simulink model "DBX_model_all"  (R2015a)
settings: Solver=ode2  SolverMode=SingleTasking  StartTime=0.0  StopTime=10  FixedStep=T_sim  RelTol=1e-3
undefined symbols (not defined in the file or in its folder): A_M, Alpha_unique_rad, as, B_span, Beta_unique_rad, C_D_q, C_l, C_l_delta_a_Asim, C_l_delta_rv_Asim, C_l_p, C_l_r, C_Lift_q, C_m, C_m_q, C_n, C_n_delta_a_Asim, C_n_delta_rv_Asim, C_n_p, C_n_r, C_X, C_Y, C_Y_delta_rv_Asim, C_Y_p, C_Y_r, C_Z, CG, CMA, DBX_aero, DBX_aero_param, delta_elev_unique_rad, DOWN_0, EAST_0, F, g, h_1, h_2, h_3, I_BAC, Initial_Omegas, Initial_Torques, Ion, L_M, Lithium, m, MIL, NORTH_0, P_0, Q_0, R_0, Rotation_sign, Servo_calib, T_sim, U_0, V_0, W_0
libraries: simulink x19, DBX_model x14, aerolibwind2 x12, aerolibasang x9, aerolibadyn x4, aerolibatmos2 x2, powerlib x2, aerolibtransform2 x1, electricdrivelib x1
(part 3 of 3)

== system DBX_model_all/Aeromodel/Aero model V2 parametric/Aerodynamics/Moment Coefficients/C_m_T ==
  note: Deflexiones del modelo Aero:
      |
      | delta_ail
      | delta_elev
      | delta_rudder
  alpha : Inport
  beta : Inport  Port=2
  body_rates_adim : Inport  Port=3  PortDimensions=[3 1]
  defl_control : Inport  Port=4
  Add : Sum  Inputs=+++|
  C_m : Subsystem
  C_m_delta_elev : Subsystem
  C_m_q : Constant  Value=DBX_aero_param.C_m_q
  Divide : Product  Inputs=**
  Selector : Selector  InputPortWidth=3  Indices=2
  Selector2 : Selector  InputPortWidth=3  Indices=2
  C_m_T : Outport
  wires:
  Add/1 -> C_m_T/1
  C_m/1(C_m_out) -> Add/1
  Divide/1 -> Add/3
  defl_control/1 -> Selector2/1
  body_rates_adim/1 -> Selector/1
  C_m_q/1 -> Divide/2
  Selector/1 -> Divide/1
  beta/1 -> C_m/2(y)
  alpha/1 -> C_m_delta_elev/1(x), C_m/1(x)
  Selector2/1 -> C_m_delta_elev/2(y)
  C_m_delta_elev/1(C_m_delta_elev_out) -> Add/2

== system DBX_model_all/Aeromodel/Aero model V2 parametric/Aerodynamics/Moment Coefficients/C_n_T ==
  note: Deflexiones del modelo Aero:
      |
      | delta_ail
      | delta_elev
      | delta_rudder
  alpha : Inport
  beta : Inport  Port=2
  body_rates_adim : Inport  Port=3  PortDimensions=[3 1]
  defl_control : Inport  Port=4
  Add : Sum  Inputs=+++++
  C_n : Subsystem
  C_n_delta_a : Constant  Value=DBX_aero_param.C_n_delta_ale
  C_n_delta_rudd : Constant  Value=DBX_aero_param.C_n_delta_rud
  C_n_p : Constant  Value=DBX_aero_param.C_n_p
  C_n_r : Constant  Value=DBX_aero_param.C_n_r
  Divide{,1..3} (4 alike) : Product  Inputs=**
  Selector : Selector  InputPortWidth=3  Indices=3
  Selector1 : Selector  InputPortWidth=3  Indices=3
  Selector2 : Selector  InputPortWidth=3
  Selector3 : Selector  InputPortWidth=3
  C_n_T : Outport
  wires:
  Divide1/1 -> Add/5
  Divide2/1 -> Add/4
  Divide3/1 -> Add/3
  Divide/1 -> Add/2
  C_n/1(C_n_out) -> Add/1
  Selector/1 -> Divide/1
  C_n_p/1 -> Divide3/2
  Selector3/1 -> Divide3/1
  body_rates_adim/1 -> Selector/1, Selector3/1
  C_n_r/1 -> Divide/2
  Selector1/1 -> Divide1/1
  C_n_delta_rudd/1 -> Divide1/2
  Selector2/1 -> Divide2/1
  C_n_delta_a/1 -> Divide2/2
  defl_control/1 -> Selector2/1, Selector1/1
  Add/1 -> C_n_T/1
  beta/1 -> C_n/2(y)
  alpha/1 -> C_n/1(x)

== system DBX_model_all/Aeromodel/Aero model V2 parametric/Aerodynamics/Wind-axes Velocities/Calculate alphadot ==
  note: W
  note: Calculate alphadot
  "[Udot Vdot Wdot]" : Inport
  "[U V W]" : Inport  Port=2
  Demux : Demux  Outputs=3
  Demux1 : Demux  Outputs=3
  Math Function : Math  Operator=square  SaturateOnIntegerOverflow=on
  Math Function1 : Math  Operator=square  SaturateOnIntegerOverflow=on
  Product : Product  RndMeth=Zero
  Product1 : Product  RndMeth=Zero
  Product2 : Product  Inputs=*/  RndMeth=Zero
  Sum : Sum  Inputs=-|+
  Sum1 : Sum  Inputs=+|+
  Terminator : Terminator
  Terminator1 : Terminator
  alphadot : Outport
  wires:
  Demux/1 -> Product1/1  "Udot"
  Demux/3 -> Product/1  "Wdot"
  Demux/2 -> Terminator/1
  Demux1/1 -> Product/2, Math Function/1  "U"
  Demux1/3 -> Product1/2, Math Function1/1
  Math Function/1 -> Sum1/1
  Math Function1/1 -> Sum1/2
  Sum1/1 -> Product2/2  "U^2 + W^2"
  Product1/1 -> Sum/1  "W Udot"
  Product/1 -> Sum/2  "U Wdot"
  Sum/1 -> Product2/1
  Demux1/2 -> Terminator1/1
  "[U V W]"/1 -> Demux1/1
  "[Udot Vdot Wdot]"/1 -> Demux/1
  Product2/1 -> alphadot/1  "alphadot"

== system DBX_model_all/Aeromodel/Aero model aerosonde/Aerodynamics/Force Coefficients/Drag Coefficients ==
  note: Drag coefficient
  control : Inport
  Mach : Inport  Port=2
  CL : Inport  Port=3  PortDimensions=1
  (CL-CL0)^2/(pi e AR) : Gain  Gain=1/as.pieaR  Multiplication=Matrix(K*u)  SaturateOnIntegerOverflow=on  OutDataTypeStr=Inherit: Same as input  ParamDataTypeStr=Inherit: Same as input
  Abs4 : Abs  SaturateOnIntegerOverflow=on
  CDM : Gain  Gain=as.CDM  SaturateOnIntegerOverflow=on  OutDataTypeStr=Inherit: Same as input  ParamDataTypeStr=Inherit: Same as input
  CDdf : Gain  Gain=[as.CDdf, as.CDde, as.CDda, as.CDdr]  Multiplication=Matrix(K*u)  SaturateOnIntegerOverflow=on  OutDataTypeStr=Inherit: Same as input  ParamDataTypeStr=Inherit: Same as input
  CL min drag : Constant  Value=as.CLmind
  CL^2 : Math  Operator=square  SaturateOnIntegerOverflow=on
  Constant terms : Constant  Value=as.CD0
  Sum : Sum  Inputs=|+-  SaturateOnIntegerOverflow=on  InputSameDT=on  OutDataTypeStr=Inherit: Same as first input
  Sum1 : Sum  Inputs=++++  SaturateOnIntegerOverflow=on  InputSameDT=on  OutDataTypeStr=Inherit: Same as first input
  CD : Outport
  wires:
  (CL-CL0)^2/(pi e AR)/1 -> Sum1/4
  CL min drag/1 -> Sum/2
  CL/1 -> Sum/1
  Sum/1 -> CL^2/1
  CL^2/1 -> (CL-CL0)^2/(pi e AR)/1
  Sum1/1 -> CD/1  "CD"
  Mach/1 -> CDM/1
  control/1 -> Abs4/1
  Abs4/1 -> CDdf/1
  CDM/1 -> Sum1/3
  CDdf/1 -> Sum1/2
  Constant terms/1 -> Sum1/1

== system DBX_model_all/Aeromodel/Aero model aerosonde/Aerodynamics/Force Coefficients/Lift Coefficients ==
  note: Lift Coefficients
  alpha : Inport
  control : Inport  Port=2
  alphadot : Inport  Port=3
  pqr : Inport  Port=4
  2V_a : Inport  Port=5
  Mach : Inport  Port=6
  CL*c/(2V_a) : Product  Inputs=*/  SaturateOnIntegerOverflow=on  InputSameDT=on  OutDataTypeStr=Inherit: Same as first input
  CL0 : Constant  Value=as.CL0
  CLM : Gain  Gain=as.CLM  SaturateOnIntegerOverflow=on  OutDataTypeStr=Inherit: Same as input  ParamDataTypeStr=Inherit: Same as input
  CLalpha : Gain  Gain=as.CLalpha  SaturateOnIntegerOverflow=on  OutDataTypeStr=Inherit: Same as input  ParamDataTypeStr=Inherit: Same as input
  CLalphadot : Gain  Gain=as.CLalphadot  Multiplication=Matrix(K*u)  SaturateOnIntegerOverflow=on  OutDataTypeStr=Inherit: Same as input  ParamDataTypeStr=Inherit: Same as input
  CLq : Gain  Gain=[0, as.CLq, 0]  Multiplication=Matrix(K*u)  SaturateOnIntegerOverflow=on  OutDataTypeStr=Inherit: Same as input  ParamDataTypeStr=Inherit: Same as input
  Sum : Sum  SaturateOnIntegerOverflow=on  InputSameDT=on  OutDataTypeStr=Inherit: Same as first input
  Sum2 : Sum  Inputs=+++++  SaturateOnIntegerOverflow=on  InputSameDT=on  OutDataTypeStr=Inherit: Same as first input
  "[CLdf, CLde, 0, 0]" : Gain  Gain=[as.CLdf, as.CLde, 0, 0]  Multiplication=Matrix(K*u)  SaturateOnIntegerOverflow=on  OutDataTypeStr=Inherit: Same as input  ParamDataTypeStr=Inherit: Same as input
  c : Gain  Gain=as.c  SaturateOnIntegerOverflow=on  OutDataTypeStr=Inherit: Same as input  ParamDataTypeStr=Inherit: Same as input
  CL : Outport
  wires:
  alphadot/1 -> CLalphadot/1
  alpha/1 -> CLalpha/1
  Mach/1 -> CLM/1
  2V_a/1 -> CL*c/(2V_a)/2
  pqr/1 -> CLq/1
  control/1 -> "[CLdf, CLde, 0, 0]"/1
  c/1 -> CL*c/(2V_a)/1
  CL*c/(2V_a)/1 -> Sum2/4
  CLM/1 -> Sum2/5
  Sum2/1 -> CL/1  "CL"
  "[CLdf, CLde, 0, 0]"/1 -> Sum2/3
  CLalpha/1 -> Sum2/2
  CL0/1 -> Sum2/1
  Sum/1 -> c/1
  CLalphadot/1 -> Sum/1
  CLq/1 -> Sum/2

== system DBX_model_all/Aeromodel/Aero model aerosonde/Aerodynamics/Force Coefficients/Side Force Coefficients ==
  note: Side force coefficients
  beta : Inport
  control : Inport  Port=2
  angular rates : Inport  Port=3
  2V_a : Inport  Port=4
  CY*b/(2V_a) : Product  Inputs=*/  SaturateOnIntegerOverflow=on  InputSameDT=on  OutDataTypeStr=Inherit: Same as first input
  CYbeta : Gain  Gain=as.CYbeta  SaturateOnIntegerOverflow=on  OutDataTypeStr=Inherit: Same as input  ParamDataTypeStr=Inherit: Same as input
  Sum3 : Sum  Inputs=+++  SaturateOnIntegerOverflow=on  InputSameDT=on  OutDataTypeStr=Inherit: Same as first input
  Wing span1 : Gain  Gain=as.b  SaturateOnIntegerOverflow=on  OutDataTypeStr=Inherit: Same as input  ParamDataTypeStr=Inherit: Same as input
  "[0, 0, CYda, CYdr]" : Gain  Gain=[0, 0, as.CYda, as.CYdr]  Multiplication=Matrix(K*u)  SaturateOnIntegerOverflow=on  OutDataTypeStr=Inherit: Same as input  ParamDataTypeStr=Inherit: Same as input
  "[CYp, 0, CYr]" : Gain  Gain=[as.CYp, 0, as.CYr]  Multiplication=Matrix(K*u)  SaturateOnIntegerOverflow=on  OutDataTypeStr=Inherit: Same as input  ParamDataTypeStr=Inherit: Same as input
  CY : Outport
  wires:
  beta/1 -> CYbeta/1
  2V_a/1 -> CY*b/(2V_a)/2
  angular rates/1 -> "[CYp, 0, CYr]"/1
  control/1 -> "[0, 0, CYda, CYdr]"/1
  Wing span1/1 -> CY*b/(2V_a)/1
  Sum3/1 -> CY/1  "CY"
  CY*b/(2V_a)/1 -> Sum3/3
  "[0, 0, CYda, CYdr]"/1 -> Sum3/2
  CYbeta/1 -> Sum3/1
  "[CYp, 0, CYr]"/1 -> Wing span1/1

== system DBX_model_all/Aeromodel/Aero model aerosonde/Aerodynamics/Moment Coefficients/Pitch Moment Coefficients ==
  alpha : Inport
  control : Inport  Port=2
  alphadot : Inport  Port=3
  pqr : Inport  Port=4
  2V_a : Inport  Port=5
  Mach : Inport  Port=6
  CMalpha : Gain  Gain=as.Cmalpha  SaturateOnIntegerOverflow=on  OutDataTypeStr=Inherit: Same as input  ParamDataTypeStr=Inherit: Same as input
  Cm*c/(2V_a) : Product  Inputs=*/  SaturateOnIntegerOverflow=on  InputSameDT=on  OutDataTypeStr=Inherit: Same as first input
  Cm0 : Constant  Value=as.Cm0
  CmM : Gain  Gain=as.CmM  SaturateOnIntegerOverflow=on  OutDataTypeStr=Inherit: Same as input  ParamDataTypeStr=Inherit: Same as input
  Cmalphadot : Gain  Gain=as.Cmalphadot  Multiplication=Matrix(K*u)  SaturateOnIntegerOverflow=on  OutDataTypeStr=Inherit: Same as input  ParamDataTypeStr=Inherit: Same as input
  Cmq : Gain  Gain=[0, as.Cmq, 0]  Multiplication=Matrix(K*u)  SaturateOnIntegerOverflow=on  OutDataTypeStr=Inherit: Same as input  ParamDataTypeStr=Inherit: Same as input
  Sum : Sum  SaturateOnIntegerOverflow=on  InputSameDT=on  OutDataTypeStr=Inherit: Same as first input
  Sum2 : Sum  Inputs=+++++  SaturateOnIntegerOverflow=on  InputSameDT=on  OutDataTypeStr=Inherit: Same as first input
  "[Cmdf, Cmde, 0, 0]" : Gain  Gain=[as.Cmdf, as.Cmde, 0, 0]  Multiplication=Matrix(K*u)  SaturateOnIntegerOverflow=on  OutDataTypeStr=Inherit: Same as input  ParamDataTypeStr=Inherit: Same as input
  c : Gain  Gain=as.c  SaturateOnIntegerOverflow=on  OutDataTypeStr=Inherit: Same as input  ParamDataTypeStr=Inherit: Same as input
  Cm : Outport
  wires:
  Cmq/1 -> Sum/2
  Cmalphadot/1 -> Sum/1
  Sum/1 -> c/1
  Cm0/1 -> Sum2/1
  CMalpha/1 -> Sum2/2
  "[Cmdf, Cmde, 0, 0]"/1 -> Sum2/3
  Sum2/1 -> Cm/1  "Cm"
  CmM/1 -> Sum2/5
  Cm*c/(2V_a)/1 -> Sum2/4
  c/1 -> Cm*c/(2V_a)/1
  control/1 -> "[Cmdf, Cmde, 0, 0]"/1
  pqr/1 -> Cmq/1
  2V_a/1 -> Cm*c/(2V_a)/2
  Mach/1 -> CmM/1
  alpha/1 -> CMalpha/1
  alphadot/1 -> Cmalphadot/1

== system DBX_model_all/Aeromodel/Aero model aerosonde/Aerodynamics/Moment Coefficients/Roll Moment Coefficients ==
  note: Roll moment coefficient
  beta : Inport
  control : Inport  Port=2
  angular rates : Inport  Port=3
  2V : Inport  Port=4
  CY*b/(2V) : Product  Inputs=*/  SaturateOnIntegerOverflow=on  InputSameDT=on  OutDataTypeStr=Inherit: Same as first input
  Clbeta : Gain  Gain=as.Clbeta  SaturateOnIntegerOverflow=on  OutDataTypeStr=Inherit: Same as input  ParamDataTypeStr=Inherit: Same as input
  Sum3 : Sum  Inputs=+++  SaturateOnIntegerOverflow=on  InputSameDT=on  OutDataTypeStr=Inherit: Same as first input
  Wing span : Gain  Gain=as.b  SaturateOnIntegerOverflow=on  OutDataTypeStr=Inherit: Same as input  ParamDataTypeStr=Inherit: Same as input
  "[0, 0, Clda, Cldr]" : Gain  Gain=[0, 0, as.Clda, as.Cldr]  Multiplication=Matrix(K*u)  SaturateOnIntegerOverflow=on  OutDataTypeStr=Inherit: Same as input  ParamDataTypeStr=Inherit: Same as input
  "[Clp, 0, Clr]" : Gain  Gain=[as.Clp, 0, as.Clr]  Multiplication=Matrix(K*u)  SaturateOnIntegerOverflow=on  OutDataTypeStr=Inherit: Same as input  ParamDataTypeStr=Inherit: Same as input
  Cl : Outport
  wires:
  "[Clp, 0, Clr]"/1 -> Wing span/1
  Clbeta/1 -> Sum3/1
  "[0, 0, Clda, Cldr]"/1 -> Sum3/2
  CY*b/(2V)/1 -> Sum3/3
  Sum3/1 -> Cl/1  "Cl"
  Wing span/1 -> CY*b/(2V)/1
  control/1 -> "[0, 0, Clda, Cldr]"/1
  angular rates/1 -> "[Clp, 0, Clr]"/1
  2V/1 -> CY*b/(2V)/2
  beta/1 -> Clbeta/1

== system DBX_model_all/Aeromodel/Aero model aerosonde/Aerodynamics/Moment Coefficients/Yaw Moment Coefficients ==
  note: Yaw moment coefficient
  beta : Inport
  control : Inport  Port=2
  angular rates : Inport  Port=3
  2V_a : Inport  Port=4
  Cn*b/(2V_a) : Product  Inputs=*/  SaturateOnIntegerOverflow=on  InputSameDT=on  OutDataTypeStr=Inherit: Same as first input
  Cnbeta : Gain  Gain=as.Cnbeta  SaturateOnIntegerOverflow=on  OutDataTypeStr=Inherit: Same as input  ParamDataTypeStr=Inherit: Same as input
  Sum3 : Sum  Inputs=+++  SaturateOnIntegerOverflow=on  InputSameDT=on  OutDataTypeStr=Inherit: Same as first input
  Wing span : Gain  Gain=as.b  SaturateOnIntegerOverflow=on  OutDataTypeStr=Inherit: Same as input  ParamDataTypeStr=Inherit: Same as input
  "[0, 0, Cnda, Cndr]" : Gain  Gain=[0, 0, as.Cnda, as.Cndr]  Multiplication=Matrix(K*u)  SaturateOnIntegerOverflow=on  OutDataTypeStr=Inherit: Same as input  ParamDataTypeStr=Inherit: Same as input
  "[Cnp, 0, Cnr]" : Gain  Gain=[as.Cnp, 0, as.Cnr]  Multiplication=Matrix(K*u)  SaturateOnIntegerOverflow=on  OutDataTypeStr=Inherit: Same as input  ParamDataTypeStr=Inherit: Same as input
  Cn : Outport
  wires:
  beta/1 -> Cnbeta/1
  2V_a/1 -> Cn*b/(2V_a)/2
  angular rates/1 -> "[Cnp, 0, Cnr]"/1
  control/1 -> "[0, 0, Cnda, Cndr]"/1
  Wing span/1 -> Cn*b/(2V_a)/1
  Sum3/1 -> Cn/1  "Cn"
  Cn*b/(2V_a)/1 -> Sum3/3
  "[0, 0, Cnda, Cndr]"/1 -> Sum3/2
  Cnbeta/1 -> Sum3/1
  "[Cnp, 0, Cnr]"/1 -> Wing span/1

== system DBX_model_all/Aeromodel/Aero model aerosonde/Aerodynamics/Wind-axes Velocities/Calculate alphadot ==
  note: Calculate alphadot
  note: W
  "[Udot Vdot Wdot]" : Inport
  "[U V W]" : Inport  Port=2
  Demux : Demux  Outputs=3
  Demux1 : Demux  Outputs=3
  Math Function : Math  Operator=square  SaturateOnIntegerOverflow=on
  Math Function1 : Math  Operator=square  SaturateOnIntegerOverflow=on
  Product : Product  RndMeth=Zero
  Product1 : Product  RndMeth=Zero
  Product2 : Product  Inputs=*/  RndMeth=Zero
  Sum : Sum  Inputs=-|+
  Sum1 : Sum  Inputs=+|+
  Terminator : Terminator
  Terminator1 : Terminator
  alphadot : Outport
  wires:
  Product2/1 -> alphadot/1  "alphadot"
  "[Udot Vdot Wdot]"/1 -> Demux/1
  "[U V W]"/1 -> Demux1/1
  Demux1/2 -> Terminator1/1
  Sum/1 -> Product2/1
  Product/1 -> Sum/2  "U Wdot"
  Product1/1 -> Sum/1  "W Udot"
  Sum1/1 -> Product2/2  "U^2 + W^2"
  Math Function1/1 -> Sum1/2
  Math Function/1 -> Sum1/1
  Demux1/3 -> Math Function1/1, Product1/2
  Demux1/1 -> Math Function/1, Product/2  "U"
  Demux/2 -> Terminator/1
  Demux/3 -> Product/1  "Wdot"
  Demux/1 -> Product1/1  "Udot"

== system DBX_model_all/Aeromodel/Aero model V2 parametric/Aerodynamics/Force Coefficients/C_X_T/C_X ==
  x : Inport
  y : Inport  Port=2
  C_X : MATLAB Function
  Constant : Constant  Value=DBX_aero_param.C_X.a
  Constant1 : Constant  Value=DBX_aero_param.C_X.x_lim
  Constant2 : Constant  Value=DBX_aero_param.C_X.y_lim
  Demux : Demux  Outputs=2
  Demux1 : Demux  Outputs=2
  Saturation Dynamic : simulink/Discontinuities/Saturation Dynamic  OutMin=[]  OutMax=[]  OutDataTypeStr=Inherit: Same as second input  OutDataType=fixdt(1, 16)  OutScaling=2^-10  DoSatur=off
  Saturation Dynamic1 : simulink/Discontinuities/Saturation Dynamic  OutMin=[]  OutMax=[]  OutDataTypeStr=Inherit: Same as second input  OutDataType=fixdt(1, 16)  OutScaling=2^-10  DoSatur=off
  Terminator : Terminator
  Unary Minus : UnaryMinus
  C_X_out : Outport
  wires:
  Constant/1 -> C_X/3(a)
  C_X/1(C_X_out) -> C_X_out/1
  Constant2/1 -> Demux1/1
  Saturation Dynamic1/1 -> C_X/2(beta_rad)
  Demux1/1 -> Unary Minus/1, Saturation Dynamic1/1
  Saturation Dynamic/1 -> C_X/1(alpha_rad)
  x/1 -> Saturation Dynamic/2
  Constant1/1 -> Demux/1
  Demux/2 -> Saturation Dynamic/3
  y/1 -> Saturation Dynamic1/2
  Demux/1 -> Saturation Dynamic/1
  Unary Minus/1 -> Saturation Dynamic1/3
  Demux1/2 -> Terminator/1

== system DBX_model_all/Aeromodel/Aero model V2 parametric/Aerodynamics/Force Coefficients/C_X_T/C_X_delta_elev ==
  x : Inport
  y : Inport  Port=2
  C_X_delta_elev : MATLAB Function
  Constant : Constant  Value=DBX_aero_param.C_X_delta_elev.a
  Constant1 : Constant  Value=DBX_aero_param.C_X_delta_elev.x_lim
  Constant2 : Constant  Value=DBX_aero_param.C_X_delta_elev.y_lim
  Demux : Demux  Outputs=2
  Demux1 : Demux  Outputs=2
  Saturation Dynamic : simulink/Discontinuities/Saturation Dynamic  OutMin=[]  OutMax=[]  OutDataTypeStr=Inherit: Same as second input  OutDataType=fixdt(1, 16)  OutScaling=2^-10  DoSatur=off
  Saturation Dynamic1 : simulink/Discontinuities/Saturation Dynamic  OutMin=[]  OutMax=[]  OutDataTypeStr=Inherit: Same as second input  OutDataType=fixdt(1, 16)  OutScaling=2^-10  DoSatur=off
  C_X_delta_elev_out : Outport
  wires:
  Demux/1 -> Saturation Dynamic/1
  y/1 -> Saturation Dynamic1/2
  Demux/2 -> Saturation Dynamic/3
  Constant1/1 -> Demux/1
  x/1 -> Saturation Dynamic/2
  Demux1/2 -> Saturation Dynamic1/3
  Saturation Dynamic/1 -> C_X_delta_elev/1(alpha_rad)
  Demux1/1 -> Saturation Dynamic1/1
  Saturation Dynamic1/1 -> C_X_delta_elev/2(delta_elev_rad)
  Constant2/1 -> Demux1/1
  C_X_delta_elev/1(C_X_delta_elev_out) -> C_X_delta_elev_out/1
  Constant/1 -> C_X_delta_elev/3(a)

== system DBX_model_all/Aeromodel/Aero model V2 parametric/Aerodynamics/Force Coefficients/C_Y_T/C_Y ==
  x : Inport
  y : Inport  Port=2
  C_Y : MATLAB Function
  Constant : Constant  Value=DBX_aero_param.C_Y.a
  Constant1 : Constant  Value=DBX_aero_param.C_Y.x_lim
  Constant2 : Constant  Value=DBX_aero_param.C_Y.y_lim
  Demux : Demux  Outputs=2
  Demux1 : Demux  Outputs=2
  Saturation Dynamic : simulink/Discontinuities/Saturation Dynamic  OutMin=[]  OutMax=[]  OutDataTypeStr=Inherit: Same as second input  OutDataType=fixdt(1, 16)  OutScaling=2^-10  DoSatur=off
  Saturation Dynamic1 : simulink/Discontinuities/Saturation Dynamic  OutMin=[]  OutMax=[]  OutDataTypeStr=Inherit: Same as second input  OutDataType=fixdt(1, 16)  OutScaling=2^-10  DoSatur=off
  Terminator : Terminator
  Unary Minus : UnaryMinus
  C_Y_out : Outport
  wires:
  Demux/1 -> Saturation Dynamic/1
  y/1 -> Saturation Dynamic1/2
  Demux/2 -> Saturation Dynamic/3
  Constant1/1 -> Demux/1
  x/1 -> Saturation Dynamic/2
  Saturation Dynamic/1 -> C_Y/1(alpha_rad)
  Demux1/1 -> Unary Minus/1, Saturation Dynamic1/1
  Saturation Dynamic1/1 -> C_Y/2(beta_rad)
  Constant2/1 -> Demux1/1
  C_Y/1(C_Y_out) -> C_Y_out/1
  Constant/1 -> C_Y/3(a)
  Unary Minus/1 -> Saturation Dynamic1/3
  Demux1/2 -> Terminator/1

== system DBX_model_all/Aeromodel/Aero model V2 parametric/Aerodynamics/Force Coefficients/C_Z_T/C_Z ==
  x : Inport
  y : Inport  Port=2
  C_Z : MATLAB Function
  Constant : Constant  Value=DBX_aero_param.C_Z.a
  Constant1 : Constant  Value=DBX_aero_param.C_Z.x_lim
  Constant2 : Constant  Value=DBX_aero_param.C_Z.y_lim
  Demux : Demux  Outputs=2
  Demux1 : Demux  Outputs=2
  Saturation Dynamic : simulink/Discontinuities/Saturation Dynamic  OutMin=[]  OutMax=[]  OutDataTypeStr=Inherit: Same as second input  OutDataType=fixdt(1, 16)  OutScaling=2^-10  DoSatur=off
  Saturation Dynamic1 : simulink/Discontinuities/Saturation Dynamic  OutMin=[]  OutMax=[]  OutDataTypeStr=Inherit: Same as second input  OutDataType=fixdt(1, 16)  OutScaling=2^-10  DoSatur=off
  Terminator : Terminator
  Unary Minus : UnaryMinus
  C_Z_out : Outport
  wires:
  Demux/1 -> Saturation Dynamic/1
  y/1 -> Saturation Dynamic1/2
  Demux/2 -> Saturation Dynamic/3
  Constant1/1 -> Demux/1
  x/1 -> Saturation Dynamic/2
  Saturation Dynamic/1 -> C_Z/1(alpha_rad)
  Demux1/1 -> Unary Minus/1, Saturation Dynamic1/1
  Saturation Dynamic1/1 -> C_Z/2(beta_rad)
  Constant2/1 -> Demux1/1
  C_Z/1(C_Z_out) -> C_Z_out/1
  Constant/1 -> C_Z/3(a)
  Unary Minus/1 -> Saturation Dynamic1/3
  Demux1/2 -> Terminator/1

== system DBX_model_all/Aeromodel/Aero model V2 parametric/Aerodynamics/Force Coefficients/C_Z_T/C_Z_delta_elev ==
  x : Inport
  y : Inport  Port=2
  C_Z_delta_elev : MATLAB Function
  Constant : Constant  Value=DBX_aero_param.C_Z_delta_elev.a
  Constant1 : Constant  Value=DBX_aero_param.C_Z_delta_elev.x_lim
  Constant2 : Constant  Value=DBX_aero_param.C_Z_delta_elev.y_lim
  Demux : Demux  Outputs=2
  Demux1 : Demux  Outputs=2
  Saturation Dynamic : simulink/Discontinuities/Saturation Dynamic  OutMin=[]  OutMax=[]  OutDataTypeStr=Inherit: Same as second input  OutDataType=fixdt(1, 16)  OutScaling=2^-10  DoSatur=off
  Saturation Dynamic1 : simulink/Discontinuities/Saturation Dynamic  OutMin=[]  OutMax=[]  OutDataTypeStr=Inherit: Same as second input  OutDataType=fixdt(1, 16)  OutScaling=2^-10  DoSatur=off
  C_Z_delta_elev_out : Outport
  wires:
  Constant/1 -> C_Z_delta_elev/3(a)
  C_Z_delta_elev/1(C_Z_delta_elev_out) -> C_Z_delta_elev_out/1
  Constant2/1 -> Demux1/1
  Saturation Dynamic1/1 -> C_Z_delta_elev/2(delta_elev_rad)
  Demux1/1 -> Saturation Dynamic1/1
  Saturation Dynamic/1 -> C_Z_delta_elev/1(alpha_rad)
  Demux1/2 -> Saturation Dynamic1/3
  x/1 -> Saturation Dynamic/2
  Constant1/1 -> Demux/1
  Demux/2 -> Saturation Dynamic/3
  y/1 -> Saturation Dynamic1/2
  Demux/1 -> Saturation Dynamic/1

== system DBX_model_all/Aeromodel/Aero model V2 parametric/Aerodynamics/Moment Coefficients/C_l_T/C_l ==
  x : Inport
  y : Inport  Port=2
  C_l : MATLAB Function
  Constant : Constant  Value=DBX_aero_param.C_l.a
  Constant1 : Constant  Value=DBX_aero_param.C_l.x_lim
  Constant2 : Constant  Value=DBX_aero_param.C_l.y_lim
  Demux : Demux  Outputs=2
  Demux1 : Demux  Outputs=2
  Saturation Dynamic : simulink/Discontinuities/Saturation Dynamic  OutMin=[]  OutMax=[]  OutDataTypeStr=Inherit: Same as second input  OutDataType=fixdt(1, 16)  OutScaling=2^-10  DoSatur=off
  Saturation Dynamic1 : simulink/Discontinuities/Saturation Dynamic  OutMin=[]  OutMax=[]  OutDataTypeStr=Inherit: Same as second input  OutDataType=fixdt(1, 16)  OutScaling=2^-10  DoSatur=off
  Terminator : Terminator
  Unary Minus : UnaryMinus
  C_l_out : Outport
  wires:
  Demux/1 -> Saturation Dynamic/1
  y/1 -> Saturation Dynamic1/2
  Demux/2 -> Saturation Dynamic/3
  Constant1/1 -> Demux/1
  x/1 -> Saturation Dynamic/2
  Saturation Dynamic/1 -> C_l/1(alpha_rad)
  Demux1/1 -> Unary Minus/1, Saturation Dynamic1/1
  Saturation Dynamic1/1 -> C_l/2(beta_rad)
  Constant2/1 -> Demux1/1
  C_l/1(C_l_out) -> C_l_out/1
  Constant/1 -> C_l/3(a)
  Unary Minus/1 -> Saturation Dynamic1/3
  Demux1/2 -> Terminator/1

== system DBX_model_all/Aeromodel/Aero model V2 parametric/Aerodynamics/Moment Coefficients/C_m_T/C_m ==
  x : Inport
  y : Inport  Port=2
  C_m : MATLAB Function
  Constant : Constant  Value=DBX_aero_param.C_m.a
  Constant1 : Constant  Value=DBX_aero_param.C_m.x_lim
  Constant2 : Constant  Value=DBX_aero_param.C_m.y_lim
  Demux : Demux  Outputs=2
  Demux1 : Demux  Outputs=2
  Saturation Dynamic : simulink/Discontinuities/Saturation Dynamic  OutMin=[]  OutMax=[]  OutDataTypeStr=Inherit: Same as second input  OutDataType=fixdt(1, 16)  OutScaling=2^-10  DoSatur=off
  Saturation Dynamic1 : simulink/Discontinuities/Saturation Dynamic  OutMin=[]  OutMax=[]  OutDataTypeStr=Inherit: Same as second input  OutDataType=fixdt(1, 16)  OutScaling=2^-10  DoSatur=off
  Terminator : Terminator
  Unary Minus : UnaryMinus
  C_m_out : Outport
  wires:
  Demux/1 -> Saturation Dynamic/1
  y/1 -> Saturation Dynamic1/2
  Demux/2 -> Saturation Dynamic/3
  Constant1/1 -> Demux/1
  x/1 -> Saturation Dynamic/2
  Saturation Dynamic/1 -> C_m/1(alpha_rad)
  Demux1/1 -> Unary Minus/1, Saturation Dynamic1/1
  Saturation Dynamic1/1 -> C_m/2(beta_rad)
  Constant2/1 -> Demux1/1
  C_m/1(C_m_out) -> C_m_out/1
  Constant/1 -> C_m/3(a)
  Unary Minus/1 -> Saturation Dynamic1/3
  Demux1/2 -> Terminator/1

== system DBX_model_all/Aeromodel/Aero model V2 parametric/Aerodynamics/Moment Coefficients/C_m_T/C_m_delta_elev ==
  x : Inport
  y : Inport  Port=2
  C_m_delta_elev : MATLAB Function
  Constant : Constant  Value=DBX_aero_param.C_m_delta_elev.a
  Constant1 : Constant  Value=DBX_aero_param.C_m_delta_elev.x_lim
  Constant2 : Constant  Value=DBX_aero_param.C_m_delta_elev.y_lim
  Demux : Demux  Outputs=2
  Demux1 : Demux  Outputs=2
  Saturation Dynamic : simulink/Discontinuities/Saturation Dynamic  OutMin=[]  OutMax=[]  OutDataTypeStr=Inherit: Same as second input  OutDataType=fixdt(1, 16)  OutScaling=2^-10  DoSatur=off
  Saturation Dynamic1 : simulink/Discontinuities/Saturation Dynamic  OutMin=[]  OutMax=[]  OutDataTypeStr=Inherit: Same as second input  OutDataType=fixdt(1, 16)  OutScaling=2^-10  DoSatur=off
  C_m_delta_elev_out : Outport
  wires:
  Constant/1 -> C_m_delta_elev/3(a)
  C_m_delta_elev/1(C_m_delta_elev_out) -> C_m_delta_elev_out/1
  Constant2/1 -> Demux1/1
  Saturation Dynamic1/1 -> C_m_delta_elev/2(delta_elev_rad)
  Demux1/1 -> Saturation Dynamic1/1
  Saturation Dynamic/1 -> C_m_delta_elev/1(alpha_rad)
  Demux1/2 -> Saturation Dynamic1/3
  x/1 -> Saturation Dynamic/2
  Constant1/1 -> Demux/1
  Demux/2 -> Saturation Dynamic/3
  y/1 -> Saturation Dynamic1/2
  Demux/1 -> Saturation Dynamic/1

== system DBX_model_all/Aeromodel/Aero model V2 parametric/Aerodynamics/Moment Coefficients/C_n_T/C_n ==
  x : Inport
  y : Inport  Port=2
  C_n : MATLAB Function
  Constant : Constant  Value=DBX_aero_param.C_n.a
  Constant1 : Constant  Value=DBX_aero_param.C_n.x_lim
  Constant2 : Constant  Value=DBX_aero_param.C_n.y_lim
  Demux : Demux  Outputs=2
  Demux1 : Demux  Outputs=2
  Saturation Dynamic : simulink/Discontinuities/Saturation Dynamic  OutMin=[]  OutMax=[]  OutDataTypeStr=Inherit: Same as second input  OutDataType=fixdt(1, 16)  OutScaling=2^-10  DoSatur=off
  Saturation Dynamic1 : simulink/Discontinuities/Saturation Dynamic  OutMin=[]  OutMax=[]  OutDataTypeStr=Inherit: Same as second input  OutDataType=fixdt(1, 16)  OutScaling=2^-10  DoSatur=off
  Terminator : Terminator
  Unary Minus : UnaryMinus
  C_n_out : Outport
  wires:
  Demux/1 -> Saturation Dynamic/1
  y/1 -> Saturation Dynamic1/2
  Demux/2 -> Saturation Dynamic/3
  Constant1/1 -> Demux/1
  x/1 -> Saturation Dynamic/2
  Saturation Dynamic/1 -> C_n/1(alpha_rad)
  Demux1/1 -> Unary Minus/1, Saturation Dynamic1/1
  Saturation Dynamic1/1 -> C_n/2(beta_rad)
  Constant2/1 -> Demux1/1
  C_n/1(C_n_out) -> C_n_out/1
  Constant/1 -> C_n/3(a)
  Unary Minus/1 -> Saturation Dynamic1/3
  Demux1/2 -> Terminator/1

== matlab function DBX_model_all/6dof Eqs of motion/Position Eqs ==
  data: A_b output; Vb input; omega input; omega_dot input; Forces input; m input; CG input
function A_b  = PositionEqs(Vb,omega,omega_dot, Forces,m, CG)



 
A_b =  1/m*( Forces ) - cross(omega,Vb) - cross(omega, cross(omega,CG)) -cross(omega_dot,CG)  ;

== matlab function DBX_model_all/6dof Eqs of motion/Rotational eqs ==
  data: omega_dot output; omega_b input; Moments input; I_BAC input
function omega_dot  = Rotational_Eq(omega_b,Moments, I_BAC)



omega_dot =  I_BAC\( Moments - cross(omega_b,I_BAC*omega_b)  );

== matlab function DBX_model_all/6dof Eqs of motion/q_dot/Quaternion_dot ==
  data: omega_b input; q_dot output; q input
function q_dot = Quaternion_dot(omega_b,q)


q_dot = 1/2*HamiltonProduct(q,[0;omega_b]);

== matlab function DBX_model_all/Aeromodel/Aero model V2/ISA ==
  data: altitude input; rho output; T output; Ps output; a output
function [rho,T,Ps,a]= ISA_atmos(altitude)


    rho0 = 1.225; tfac = 1 - 6.5e-3/288.15*altitude;
    T = 288.15*tfac; if (altitude >= 11000) T = 216.65; end;
    rho = rho0*(tfac.^4.2586);
    Ps = 287*rho*T;
    a=sqrt(1.4*287*T);
    
end

== matlab function DBX_model_all/Aeromodel/Aero model aerosonde/ISA ==
  data: altitude input; rho output; T output; Ps output; a output
function [rho,T,Ps,a]= ISA_atmos(altitude)


    rho0 = 1.225; tfac = 1 - 6.5e-3/288.15*altitude;
    T = 288.15*tfac; if (altitude >= 11000) T = 216.65; end;
    rho = rho0*(tfac.^4.2586);
    Ps = 287*rho*T;
    a=sqrt(1.4*287*T);
    
end

== matlab function DBX_model_all/Aeromodel/Aero model V1/ISA ==
  data: altitude input; rho output; T output; Ps output; a output
function [rho,T,Ps,a]= ISA_atmos(altitude)


    rho0 = 1.225; tfac = 1 - 6.5e-3/288.15*altitude;
    T = 288.15*tfac; if (altitude >= 11000) T = 216.65; end;
    rho = rho0*(tfac.^4.2586);
    Ps = 287*rho*T;
    a=sqrt(1.4*287*T);
    
end

== matlab function DBX_model_all/Aeromodel/Aero model V2 parametric/ISA ==
  data: altitude input; rho output; T output; Ps output; a output
function [rho,T,Ps,a]= ISA_atmos(altitude)


    rho0 = 1.225; tfac = 1 - 6.5e-3/288.15*altitude;
    T = 288.15*tfac; if (altitude >= 11000) T = 216.65; end;
    rho = rho0*(tfac.^4.2586);
    Ps = 287*rho*T;
    a=sqrt(1.4*287*T);
    
end

== matlab function DBX_model_all/6dof Eqs of motion/Eccelerometer meas ==
  data: Vb input double; omega input; omega_dot input; Ab input; A_s output double; r_sens parameter
function A_s  = AcellMeas(Vb,omega,omega_dot,Ab, r_sens)




A_s =  Ab + cross(omega,Vb) + cross(omega, cross(omega,r_sens)) +cross(omega_dot,r_sens)  ;

== matlab function DBX_model_all/Aeromodel/Aero model V2 parametric/Aerodynamics/Force Coefficients/C_X_T/C_X/C_X ==
  data: alpha_rad input; beta_rad input; a input; C_X_out output
function C_X_out   = DBX_aero_C_X(alpha_rad,beta_rad,a)
%% C_X(alpha,beta) = (a(1)+a(2)*alpha_rad+a(3)*alpha_rad^2+a(4)*alpha_rad^3+a(5)*alpha_rad^4)*(1-beta_rad^2)



C_X_out     =    (a(1)+a(2)*alpha_rad+a(3)*alpha_rad^2+a(4)*alpha_rad^3+a(5)*alpha_rad^4)*(1-beta_rad^2);

end

== matlab function DBX_model_all/Aeromodel/Aero model V2 parametric/Aerodynamics/Force Coefficients/C_X_T/C_X_delta_elev/C_X_delta_elev ==
  data: alpha_rad input; delta_elev_rad input; a input; C_X_delta_elev_out output
function C_X_delta_elev_out   = DBX_aero_C_X_delta_elev(alpha_rad,delta_elev_rad,a)
% % C_X_delta_elev(alpha,delta_elev) = (a_0+a_1*alpha_rad+a_2*alpha_rad^2+a_3*alpha_rad^3+a_4*alpha_rad^4) + a_5*delta_elev_rad + a_6*delta_elev_rad^2



C_X_delta_elev_out     =    (a(1)+a(2)*alpha_rad+a(3)*alpha_rad^2+a(4)*alpha_rad^3+a(5)*alpha_rad^4) + a(6)*delta_elev_rad + a(7)*delta_elev_rad^2;

end

== matlab function DBX_model_all/6dof Eqs of motion/SVFI_to_SVFb ==
  data: X_e input; V_e input; X_e_out output; V_b output; omega_b output; Euler_Ang input; Euler_Ang_Dot input; q output
function [X_e_out,V_b, omega_b ,q]=SVFI_to_SVFb(X_e,V_e, Euler_Ang,Euler_Ang_Dot)

q = zeros(4,1);
V_b =zeros(3,1);

xp=V_e(1);
yp=V_e(2);
zp=V_e(3);

phi=Euler_Ang(1);
theta=Euler_Ang(2);
psi=Euler_Ang(3);
phip=Euler_Ang_Dot(1);
thetap=Euler_Ang_Dot(2);
psip=Euler_Ang_Dot(3);

%%
X_e_out=X_e;

q = QuaternionfromEuler(phi,theta,psi); 



HamOut=HamiltonProduct([q(1);-q(2);-q(3);-q(4)],HamiltonProduct([0;xp;yp;zp],[q(1);q(2);q(3);q(4)]) );% q* . v . q
V_b=HamOut(2:4);

omega_b=[phip-psip*sin(theta)  ;
         thetap*cos(phi)+psip*cos(theta)*sin(phi);
            -thetap*sin(phi)+psip*cos(theta)*cos(phi)  ];% Ya que es solo una operacion aislada utilizaremos la ecuaciones con rel trigonometricas

function [q]=QuaternionfromEuler(phi,theta,psi)
% options=optimset('MaxFunEvals',3000);
% q=fsolve(@QUATERNIONEULER,[0.6,0.4,0.5,0.4]); % Hay que acertar con los angulos poniendo diferentes valores iniciales del quaternion
%     function F=QUATERNIONEULER(q)
%         F=[ tan(phi)-(2*q(3)*q(4)-2*q(1)*q(2))/(2*q(1)^2+2*q(4)^2-1)  ;
%             sin(-theta)-2*q(2)*q(4)-2*q(1)*q(3);
%             tan(psi)-(2*q(2)*q(3)-2*q(1)*q(4))/(2*q(1)^2+2*q(2)^2-1);
%             q(1)^2+q(2)^2+q(3)^2+q(4)^2-1];
%     end  % Este algoritmo da q* !!!!!

q=[ cos(psi/2)*cos(theta/2)*cos(phi/2)+ sin(psi/2)*sin(theta/2)*sin(phi/2) ;
      cos(psi/2)*cos(theta/2)*sin(phi/2)- sin(psi/2)*sin(theta/2)*cos(phi/2) ;
       cos(psi/2)*sin(theta/2)*cos(phi/2)+ sin(psi/2)*cos(theta/2)*sin(phi/2)   ;
        sin(psi/2)*cos(theta/2)*cos(phi/2)- cos(psi/2)*sin(theta/2)*sin(phi/2)      ]; % Esto nos da q !!!

    function Product= HamiltonProduct( a,b )

Product=[ a(1)*b(1)-a(2)*b(2)-a(3)*b(3)-a(4)*b(4) ; a(1)*b(2)+a(2)*b(1)+a(3)*b(4)-a(4)*b(3)  ; a(1)*b(3)-a(2)*b(4)+a(3)*b(1)+a(4)*b(2)  ; a(1)*b(4)+a(2)*b(3)-a(3)*b(2)+a(4)*b(1) ];

== matlab function DBX_model_all/6dof Eqs of motion/SV_F_b_to_SV_FI ==
  data: V_b input; q_dot input; q input; V_e output; euler output; euler_dot output
function [V_e,euler,euler_dot]= SV_F_b_to_SV_FI(  V_b, q_dot,q)

xp=V_b(1);
yp=V_b(2);
zp=V_b(3);

%% Velocity and position in Earth Frame   q . v . q*

SolProd=HamiltonProduct([q(1);q(2);q(3);q(4)],HamiltonProduct([0;xp;yp;zp],[q(1);-q(2);-q(3);-q(4)]) );
V_e=SolProd(2:4);

%% Actitud en Angulos de Euler y sus derivadas. 
euler=[0,0,0]';
euler(1,1) = atan2(2*q(3)*q(4)+2*q(1)*q(2),2*q(1)^2+2*q(4)^2-1 ); % phi
euler(2,1) = -asin( 2*q(2)*q(4)-2*q(1)*q(3) ); %  theta
euler(3,1) = atan2( 2*q(2)*q(3)+2*q(1)*q(4),2*q(1)^2+2*q(2)^2-1 ); %  psi

euler_dot=[0,0,0]';
euler_dot(1,1) = 2/(1+( (2*q(3)*q(4)+2*q(1)*q(2))/(2*q(1)^2+2*q(4)^2-1)  )^2)*[ -(2*q(1)^2*q(2)+ 4*q(1)*q(3)*q(4)-2*q(2)*q(4)^2+q(2))  ,  q(1)*(2*q(1)^2+2*q(4)^2-1)  ,  q(4)*(2*q(1)^2+2*q(4)^2-1)  ,  -(-2*q(1)^2*q(3) +4*q(1)*q(2)*q(4)+2*q(3)*q(4)^2+q(3) ) ]*q_dot.* 1/(2*q(1)^2+2*q(4)^2-1)^2; % Derivada de phi
euler_dot(2,1) = -2/( sqrt(1-4*(q(2)*q(4)-q(1)*q(3))^2)  )*[-q(3),q(4),-q(1),q(2)]*q_dot;  % Theta prima
euler_dot(3,1) = 2/(1+( (2*q(2)*q(3)+2*q(1)*q(4))/(2*q(1)^2+2*q(2)^2-1)  )^2)*[  -(2*q(1)^2*q(4)+4*q(1)*q(2)*q(3)-2*q(2)^2*q(4)+q(4)  ) , 1/2*(q(3)*(4*q(1)^2-4*q(2)^2-2)-8*q(1)*q(2)*q(4) )  ,  q(2)*(2*q(1)^2+2*q(2)^2-1)  , q(1)*(2*q(1)^2+2*q(2)^2-1) ]*q_dot.*1/(2*q(1)^2+2*q(2)^2-1)^2;  % Psi prima

end
function Product= HamiltonProduct( a,b )

Product=[ a(1)*b(1)-a(2)*b(2)-a(3)*b(3)-a(4)*b(4) ; a(1)*b(2)+a(2)*b(1)+a(3)*b(4)-a(4)*b(3)  ; a(1)*b(3)-a(2)*b(4)+a(3)*b(1)+a(4)*b(2)  ; a(1)*b(4)+a(2)*b(3)-a(3)*b(2)+a(4)*b(1) ];
end

== matlab function DBX_model_all/Aeromodel/Aero model V2 parametric/Aerodynamics/Force Coefficients/C_Y_T/C_Y/C_Y ==
  data: alpha_rad input; beta_rad input; a input; C_Y_out output
function C_Y_out   = DBX_aero_C_Y(alpha_rad,beta_rad,a)
%% C_Y(alpha,beta) = a_1*beta_rad + a_2*alpha_rad + a_3*beta_rad^2 + a_4*alpha_rad^2 + a_5*alpha_rad*beta_rad


C_Y_out     =    a(1)*beta_rad + a(2)*alpha_rad + a(3)*beta_rad^2 + a(4)*alpha_rad^2 + a(5)*alpha_rad*beta_rad;

end

== matlab function DBX_model_all/Aeromodel/Aero model V2 parametric/Aerodynamics/Force Coefficients/C_Z_T/C_Z/C_Z ==
  data: alpha_rad input; beta_rad input; a input; C_Z_out output
function C_Z_out   = DBX_aero_C_Z(alpha_rad,beta_rad,a)
%% C_Z(alpha,beta) = (a(1)+a(2)*alpha_rad+a(3)*alpha_rad^2+a(4)*alpha_rad^3+a(5)*alpha_rad^4)*(1-beta_rad^2)



C_Z_out     =    (a(1)+a(2)*alpha_rad+a(3)*alpha_rad^2+a(4)*alpha_rad^3+a(5)*alpha_rad^4)*(1-beta_rad^2);

end

== matlab function DBX_model_all/Aeromodel/Aero model V2 parametric/Aerodynamics/Force Coefficients/C_Z_T/C_Z_delta_elev/C_Z_delta_elev ==
  data: alpha_rad input; delta_elev_rad input; a input; C_Z_delta_elev_out output
function C_Z_delta_elev_out   = DBX_aero_C_Z_delta_elev(alpha_rad,delta_elev_rad,a)
% % C_Z_delta_elev(alpha,delta_elev) = (a_0+a_1*alpha_rad+a_2*alpha_rad^2+a_3*alpha_rad^3+a_4*alpha_rad^4) + a_5*delta_elev_rad + a_6*delta_elev_rad^2



C_Z_delta_elev_out     =    (a(1)+a(2)*alpha_rad+a(3)*alpha_rad^2+a(4)*alpha_rad^3+a(5)*alpha_rad^4) + a(6)*delta_elev_rad + a(7)*delta_elev_rad^2;

end

== matlab function DBX_model_all/Aeromodel/Aero model V2 parametric/Aerodynamics/Moment Coefficients/C_l_T/C_l/C_l ==
  data: alpha_rad input; beta_rad input; a input; C_l_out output
function C_l_out   = DBX_aero_C_l(alpha_rad,beta_rad,a)
%% C_l(alpha,beta) =  a_1*beta_rad+a_2*beta_rad*alpha_rad+a_3*alpha_rad^2*beta_rad+a_4*beta_rad^2+a_5*alpha_rad*beta_rad^2+a_6*alpha_rad^3*beta_rad+a_7*alpha_rad^4*beta_rad+a_8*alpha_rad^2*beta_rad^2


C_l_out     =     a(1)*beta_rad+a(2)*beta_rad*alpha_rad+a(3)*alpha_rad^2*beta_rad+a(4)*beta_rad^2+a(5)*alpha_rad*beta_rad^2+a(6)*alpha_rad^3*beta_rad+a(7)*alpha_rad^4*beta_rad+a(8)*alpha_rad^2*beta_rad^2;

end

== matlab function DBX_model_all/Aeromodel/Aero model V2 parametric/Aerodynamics/Moment Coefficients/C_m_T/C_m/C_m ==
  data: alpha_rad input; beta_rad input; a input; C_m_out output
function C_m_out   = DBX_aero_C_m(alpha_rad,beta_rad,a)
%% C_m(alpha,beta) = (a(1)+a(2)*alpha_rad+a(3)*alpha_rad^2+a(4)*alpha_rad^3+a(5)*alpha_rad^4)*(1-beta_rad^2)

C_m_out     =    (a(1)+a(2)*alpha_rad+a(3)*alpha_rad^2+a(4)*alpha_rad^3+a(5)*alpha_rad^4)*(1-beta_rad^2);

end

== matlab function DBX_model_all/Aeromodel/Aero model V2 parametric/Aerodynamics/Moment Coefficients/C_m_T/C_m_delta_elev/C_m_delta_elev ==
  data: alpha_rad input; delta_elev_rad input; a input; C_m_delta_elev_out output
function C_m_delta_elev_out   = DBX_aero_C_m_delta_elev(alpha_rad,delta_elev_rad,a)
% %  C_m_delta_elev(alpha,delta_elev) = a_1*alpha_rad+a_2*delta_elev_rad+a_3*alpha_rad*delta_elev_rad+a_4*delta_elev_rad^2+a_5*alpha_rad^2*delta_elev_rad+a_6*delta_elev_rad^3+a_7*alpha_rad*delta_elev_rad^2

C_m_delta_elev_out     =     a(1)*alpha_rad+a(2)*delta_elev_rad+a(3)*alpha_rad*delta_elev_rad+a(4)*delta_elev_rad^2+a(5)*alpha_rad^2*delta_elev_rad+a(6)*delta_elev_rad^3+a(7)*alpha_rad*delta_elev_rad^2 ; 

end

== matlab function DBX_model_all/Aeromodel/Aero model V2 parametric/Aerodynamics/Moment Coefficients/C_n_T/C_n/C_n ==
  data: alpha_rad input; beta_rad input; a input; C_n_out output
function C_n_out   = DBX_aero_C_n(alpha_rad,beta_rad,a)
%% C_n(alpha,beta) =   a_1*beta_rad+a_2*beta_rad*alpha_rad+a_3*alpha_rad^2*beta_rad+a_4*beta_rad^2+a_5*alpha_rad*beta_rad^2+a_6*alpha_rad^3*beta_rad+a_7*alpha_rad^4*beta_rad+a_8*alpha_rad^2*beta_rad^2


C_n_out     =      a(1)*beta_rad+a(2)*beta_rad*alpha_rad+a(3)*alpha_rad^2*beta_rad+a(4)*beta_rad^2+a(5)*alpha_rad*beta_rad^2+a(6)*alpha_rad^3*beta_rad+a(7)*alpha_rad^4*beta_rad+a(8)*alpha_rad^2*beta_rad^2;

end
